simulink model "dynamicCalibrationDataGenerator"  (R2022b)
settings: Solver=VariableStepAuto  StartTime=0.0  StopTime=20  RelTol=1e-3
values from neighbouring files (symbols this model uses):
  acc_bias = [2*(rand-0.5)*acc_xy_bias_tolerance 2*(rand-0.5)*acc_xy_bias_tolerance 2*(rand-0.5)*acc_z_bias_tolerance]    [sim_cfg.m]
  acc_bias_over_temp = 2*(rand([1 3])-0.5)*acc_bias_over_temp_tolerance    [sim_cfg.m]
  acc_dynamic = 2*9.81    (= 19.62)    [sim_cfg.m]
  acc_freq = 100    [sim_cfg.m]
  acc_gain_over_temp = diag(2*(rand([1 3])-0.5)*acc_bias_over_temp_tolerance)    [sim_cfg.m]
  acc_noise = 0.008*9.81    (= 0.07848)    [sim_cfg.m]
  acc_non_orthogonality = acc_axis_alignement*acc_non_orthogonality    [sim_cfg.m]
  f_sim = 100    [sim_cfg.m]
  gps_freq = 20    [sim_cfg.m]
  gps_xy_noise = 0.1    [sim_cfg.m]
  gps_z_noise = 0.1    [sim_cfg.m]
  gravity = 9.81+rand()*0.005    [sim_cfg.m]
  gyr_bias = 2*(rand([1 3])-0.5)*gyr_bias_tolerance    [sim_cfg.m]
  gyr_bias_over_temp = 2*(rand([1 3])-0.5)*gyr_bias_over_temp_tolerance    [sim_cfg.m]
  gyr_dynamic = 250*pi/180    (= 4.36332312999)    [sim_cfg.m]
  gyr_freq = 100    [sim_cfg.m]
  gyr_gain_over_temp = diag(2*(rand([1 3])-0.5)*gyr_bias_over_temp_tolerance)    [sim_cfg.m]
  gyr_noise = 0.1*pi/180    (= 0.00174532925199)    [sim_cfg.m]
  gyr_non_orthogonality = gyr_axis_alignement*gyr_non_orthogonality    [sim_cfg.m]
  random_move_power = 3    [sim_cfg.m]
  temp_dynamic = 1    [sim_cfg.m]
libraries: simulink x10
settings Model: Creator=student  LastModifiedBy=robin

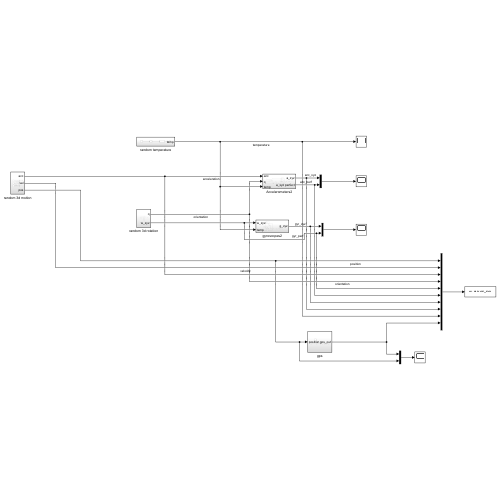
[thumbnail: Simulink's stored preview of the top-level diagram]
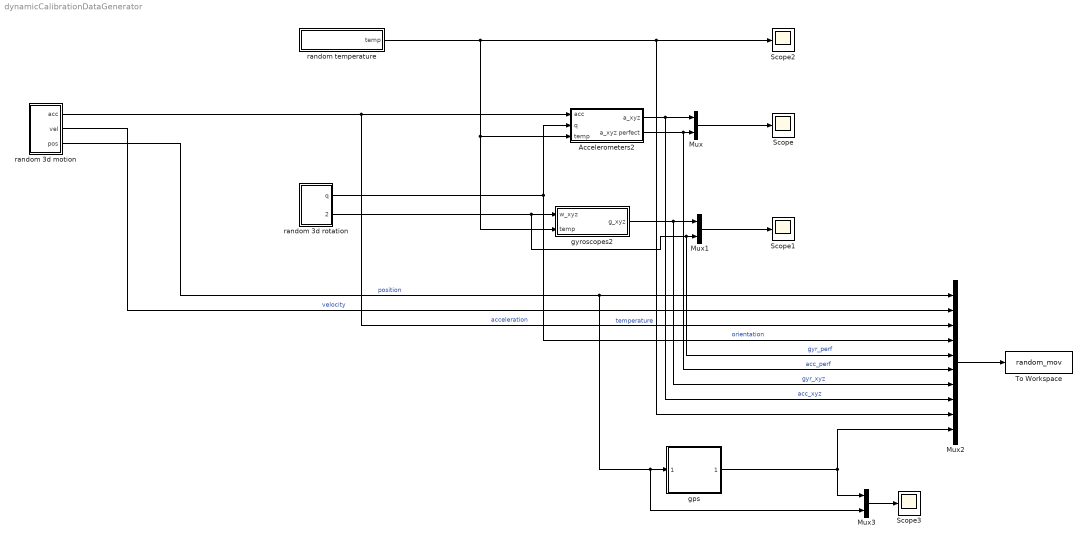
== system dynamicCalibrationDataGenerator ==
  Accelerometers2 : Subsystem
  Mux : Mux  Inputs=2
  Mux1 : Mux  Inputs=2
  Mux2 : Mux  Inputs=10
  Mux3 : Mux  Inputs=2
  Scope{,1..3} (4 alike) : Scope
  To Workspace : ToWorkspace  VariableName=random_mov  SaveFormat=Structure With Time  SampleTime=1/f_sim
  gps : Subsystem
  gyroscopes2 : Subsystem
  random 3d motion : Subsystem
  random 3d rotation : Subsystem
  random temperature : Subsystem
  wires:
  random 3d motion/1(acc) -> Accelerometers2/1(acc), Mux2/3  "acceleration"
  random 3d rotation/1(q) -> Accelerometers2/2(q), Mux2/4  "orientation"
  random 3d rotation/2(w_xyz) -> gyroscopes2/1(w_xyz), Mux2/5, Mux1/2  "gyr_perf"
  gyroscopes2/1(g_xyz) -> Mux2/7, Mux1/1  "gyr_xyz"
  random temperature/1(temp) -> gyroscopes2/2(temp), Accelerometers2/3(temp), Scope2/1, Mux2/9  "temperature"
  Accelerometers2/1(a_xyz) -> Mux2/8, Mux/1  "acc_xyz"
  Accelerometers2/2(a_xyz perfect) -> Mux2/6, Mux/2  "acc_perf"
  Mux/1 -> Scope/1
  Mux1/1 -> Scope1/1
  random 3d motion/3(pos) -> Mux3/2, gps/1(position), Mux2/1  "position"
  random 3d motion/2(vel) -> Mux2/2  "velocity"
  Mux2/1 -> To Workspace/1
  gps/1(gps_out) -> Mux3/1, Mux2/10
  Mux3/1 -> Scope3/1

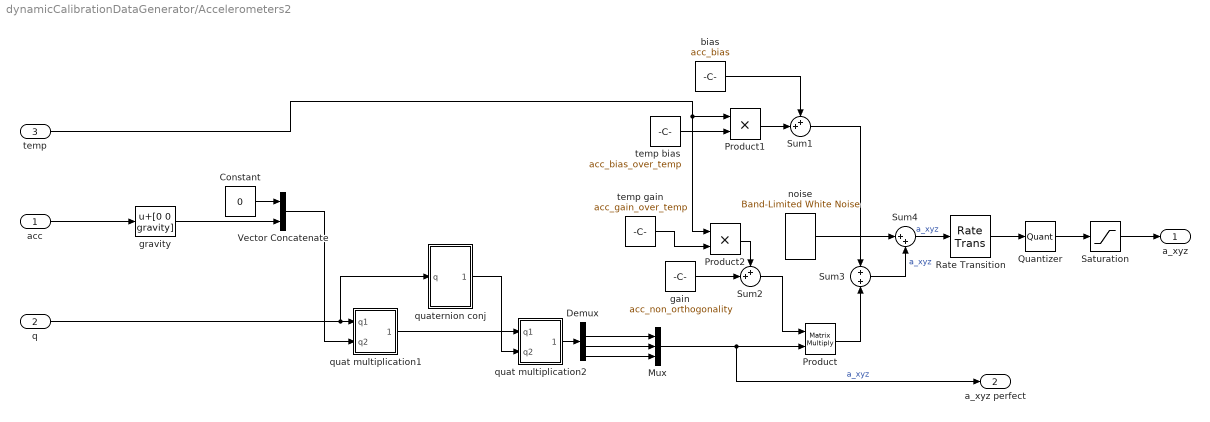
== system dynamicCalibrationDataGenerator/Accelerometers2 ==
  acc : Inport
  q : Inport  Port=2
  temp : Inport  Port=3
  Constant : Constant  Value=0
  Demux : Demux
  Mux : Mux  Inputs=3
  Product : Product  Multiplication=Matrix(*)
  Product1 : Product
  Product2 : Product
  Quantizer : Quantizer  QuantizationInterval=acc_res
  Rate Transition : RateTransition  OutPortSampleTime=1/acc_freq
  Saturation : Saturate  UpperLimit=acc_dynamic  LowerLimit=-acc_dynamic
  Sum1 : Sum  Inputs=++|
  Sum2 : Sum  Inputs=++|
  Sum3 : Sum
  Sum4 : Sum  Inputs=|++
  Vector Concatenate : Concatenate
  bias : Constant  Value=acc_bias
  gain : Constant  Value=acc_non_orthogonality
  gravity : Bias  Bias=[0 0 gravity]  SaturateOnIntegerOverflow=off
  noise : simulink/Sources/Band-Limited White Noise  Cov=[2*(2*pi*acc_noise/acc_freq)^2 2*(2*pi*acc_noise/acc_freq)^2 2*(2*pi*acc_noise/acc_freq)^2]  Ts=1/acc_freq  seed=[randi(10000) randi(10000) randi(10000)]  VectorParams1D=off
  quat multiplication1 : Subsystem
  quat multiplication2 : Subsystem
  quaternion conj : Subsystem
  temp bias : Constant  Value=acc_bias_over_temp
  temp gain : Constant  Value=acc_gain_over_temp
  a_xyz : Outport
  a_xyz perfect : Outport  Port=2
  wires:
  q/1 -> quat multiplication1/1(q1), quaternion conj/1(q)
  Sum4/1 -> Rate Transition/1  "a_xyz"
  Constant/1 -> Vector Concatenate/1
  Vector Concatenate/1 -> quat multiplication1/2(q2)
  gravity/1 -> Vector Concatenate/2
  quaternion conj/1(q conj) -> quat multiplication2/2(q2)
  quat multiplication1/1(q1*q2) -> quat multiplication2/1(q1)
  acc/1 -> gravity/1
  quat multiplication2/1(q1*q2) -> Demux/1
  Demux/2 -> Mux/1
  Demux/3 -> Mux/2
  Demux/4 -> Mux/3
  bias/1 -> Sum1/1
  Product1/1 -> Sum1/2
  temp bias/1 -> Product1/2
  temp/1 -> Product2/1, Product1/1
  temp gain/1 -> Product2/2
  gain/1 -> Sum2/2
  Sum2/1 -> Product/1
  Product2/1 -> Sum2/1
  Product/1 -> Sum3/2
  Sum1/1 -> Sum3/1
  Sum3/1 -> Sum4/2  "a_xyz"
  noise/1 -> Sum4/1
  Mux/1 -> a_xyz perfect/1, Product/2  "a_xyz"
  Saturation/1 -> a_xyz/1
  Rate Transition/1 -> Quantizer/1
  Quantizer/1 -> Saturation/1

== system dynamicCalibrationDataGenerator/gps ==
  position : Inport
  Band-Limited White Noise1 : simulink/Sources/Band-Limited White Noise  Cov=[2*(2*pi*gps_xy_noise/gps_freq)^2 2*(2*pi*gps_xy_noise/gps_freq)^2 2*(2*pi*gps_z_noise/gps_freq)^2]  Ts=1/gps_freq  seed=[randi(10000) randi(10000) randi(10000)]  VectorParams1D=off
  Quantizer : Quantizer  QuantizationInterval=gps_res
  Rate Transition : RateTransition  OutPortSampleTime=1/gps_freq
  Sum3 : Sum  Inputs=++|
  gps_out : Outport
  wires:
  Rate Transition/1 -> Quantizer/1
  Quantizer/1 -> gps_out/1
  Band-Limited White Noise1/1 -> Sum3/1
  Sum3/1 -> Rate Transition/1
  position/1 -> Sum3/2

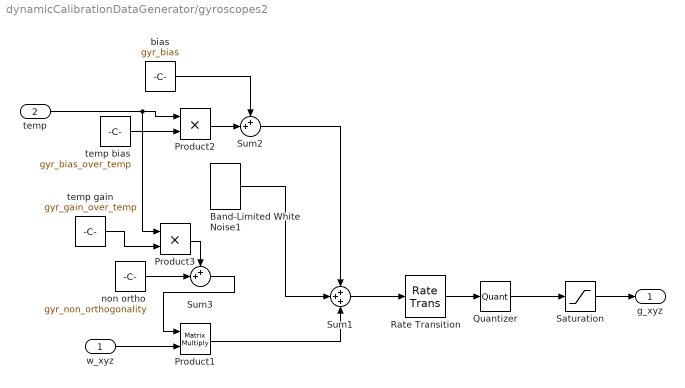
== system dynamicCalibrationDataGenerator/gyroscopes2 ==
  w_xyz : Inport
  temp : Inport  Port=2
  Band-Limited White Noise1 : simulink/Sources/Band-Limited White Noise  Cov=[2*(2*pi*gyr_noise/gyr_freq)^2 2*(2*pi*gyr_noise/gyr_freq)^2 2*(2*pi*gyr_noise/gyr_freq)^2]  Ts=1/gyr_freq  seed=[randi(10000) randi(10000) randi(10000)]  VectorParams1D=off
  Product1 : Product  Multiplication=Matrix(*)
  Product2 : Product
  Product3 : Product
  Quantizer : Quantizer  QuantizationInterval=gyr_res
  Rate Transition : RateTransition  OutPortSampleTime=1/gyr_freq
  Saturation : Saturate  UpperLimit=gyr_dynamic  LowerLimit=-gyr_dynamic
  Sum1 : Sum  Inputs=+++
  Sum2 : Sum  Inputs=++|
  Sum3 : Sum  Inputs=++|
  bias : Constant  Value=gyr_bias
  non ortho : Constant  Value=gyr_non_orthogonality
  temp bias : Constant  Value=gyr_bias_over_temp
  temp gain : Constant  Value=gyr_gain_over_temp
  g_xyz : Outport
  wires:
  non ortho/1 -> Sum3/2
  Product3/1 -> Sum3/1
  temp/1 -> Product3/1, Product2/1
  Product2/1 -> Sum2/2
  temp gain/1 -> Product3/2
  temp bias/1 -> Product2/2
  Sum3/1 -> Product1/1
  bias/1 -> Sum2/1
  Band-Limited White Noise1/1 -> Sum1/2
  Sum2/1 -> Sum1/1
  w_xyz/1 -> Product1/2
  Product1/1 -> Sum1/3
  Saturation/1 -> g_xyz/1
  Rate Transition/1 -> Quantizer/1
  Sum1/1 -> Rate Transition/1
  Quantizer/1 -> Saturation/1

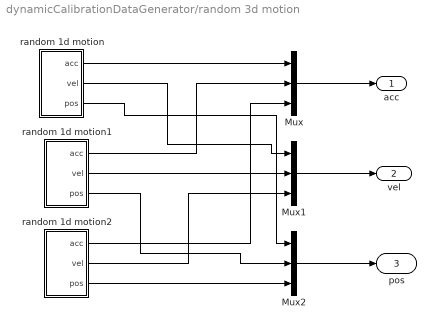
== system dynamicCalibrationDataGenerator/random 3d motion ==
  Mux : Mux  Inputs=3
  Mux1 : Mux  Inputs=3
  Mux2 : Mux  Inputs=3
  random 1d motion : Subsystem
  random 1d motion1 : Subsystem
  random 1d motion2 : Subsystem
  acc : Outport
  vel : Outport  Port=2
  pos : Outport  Port=3
  wires:
  random 1d motion/2(vel) -> Mux1/1
  random 1d motion1/3(pos) -> Mux2/2
  random 1d motion1/2(vel) -> Mux1/2
  Mux/1 -> acc/1
  random 1d motion/3(pos) -> Mux2/1
  random 1d motion2/3(pos) -> Mux2/3
  random 1d motion2/2(vel) -> Mux1/3
  random 1d motion2/1(acc) -> Mux/3
  random 1d motion/1(acc) -> Mux/1
  random 1d motion1/1(acc) -> Mux/2
  Mux1/1 -> vel/1
  Mux2/1 -> pos/1

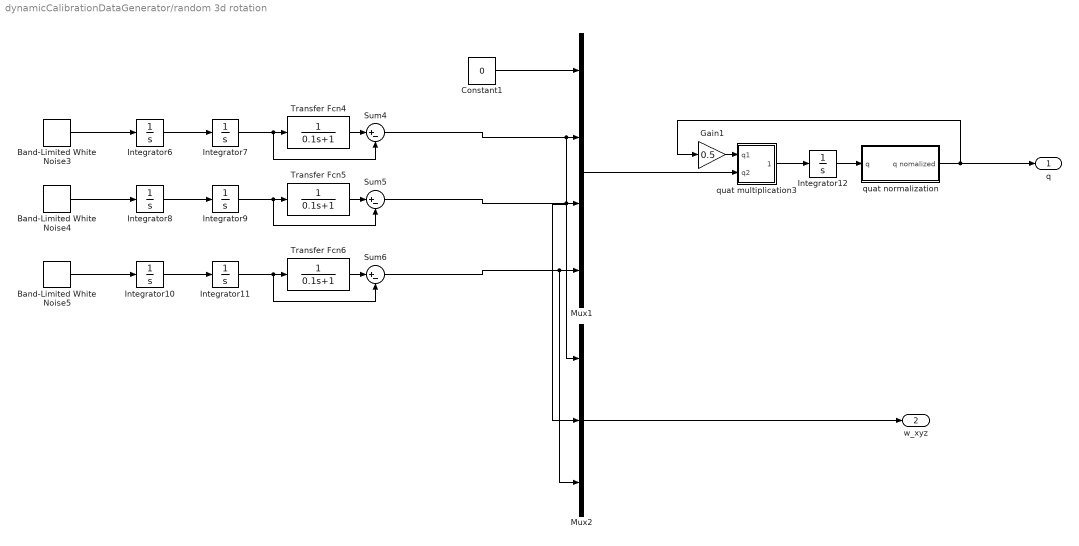
== system dynamicCalibrationDataGenerator/random 3d rotation ==
  Band-Limited White Noise3 : simulink/Sources/Band-Limited White Noise  Cov=[1]  Ts=0.1  seed=[randi(10000)]
  Band-Limited White Noise4 : simulink/Sources/Band-Limited White Noise  Cov=[1]  Ts=0.1  seed=[randi(10000)]
  Band-Limited White Noise5 : simulink/Sources/Band-Limited White Noise  Cov=[1]  Ts=0.1  seed=[randi(10000)]
  Constant1 : Constant  Value=0
  Gain1 : Gain  Gain=0.5
  Integrator{6..11} (6 alike) : Integrator
  Integrator12 : Integrator  InitialCondition=[1 0 0 0]
  Mux1 : Mux
  Mux2 : Mux  Inputs=3
  Sum4 : Sum  Inputs=|+-
  Sum5 : Sum  Inputs=|+-
  Sum6 : Sum  Inputs=|+-
  Transfer Fcn4 : TransferFcn  Denominator=[0.1 1]
  Transfer Fcn5 : TransferFcn  Denominator=[0.1 1]
  Transfer Fcn6 : TransferFcn  Denominator=[0.1 1]
  quat multiplication3 : Subsystem
  quat normalization : Subsystem
  q : Outport
  w_xyz : Outport  Port=2
  wires:
  Sum6/1 -> Mux1/4, Mux2/3
  Gain1/1 -> quat multiplication3/1(q1)
  Constant1/1 -> Mux1/1
  Mux2/1 -> w_xyz/1
  Sum4/1 -> Mux2/1, Mux1/2
  Integrator12/1 -> quat normalization/1(q)
  Sum5/1 -> Mux2/2, Mux1/3
  Integrator6/1 -> Integrator7/1
  Transfer Fcn6/1 -> Sum6/1
  Band-Limited White Noise4/1 -> Integrator8/1
  Integrator10/1 -> Integrator11/1
  Integrator7/1 -> Sum4/2, Transfer Fcn4/1
  Band-Limited White Noise5/1 -> Integrator10/1
  Integrator11/1 -> Sum6/2, Transfer Fcn6/1
  Mux1/1 -> quat multiplication3/2(q2)
  Integrator8/1 -> Integrator9/1
  Band-Limited White Noise3/1 -> Integrator6/1
  Integrator9/1 -> Sum5/2, Transfer Fcn5/1
  Transfer Fcn4/1 -> Sum4/1
  Transfer Fcn5/1 -> Sum5/1
  quat multiplication3/1(q1*q2) -> Integrator12/1
  quat normalization/1(q nomalized) -> Gain1/1, q/1

== system dynamicCalibrationDataGenerator/random temperature ==
  Band-Limited White Noise : simulink/Sources/Band-Limited White Noise  Cov=[1]  Ts=0.1  seed=[randi(10000)]
  Integrator Limited : Integrator  LimitOutput=on  UpperSaturationLimit=temp_dynamic/2  LowerSaturationLimit=-temp_dynamic/2
  Transfer Fcn1 : TransferFcn  Denominator=[0.1 1]
  temp : Outport
  wires:
  Band-Limited White Noise/1 -> Integrator Limited/1
  Transfer Fcn1/1 -> temp/1
  Integrator Limited/1 -> Transfer Fcn1/1

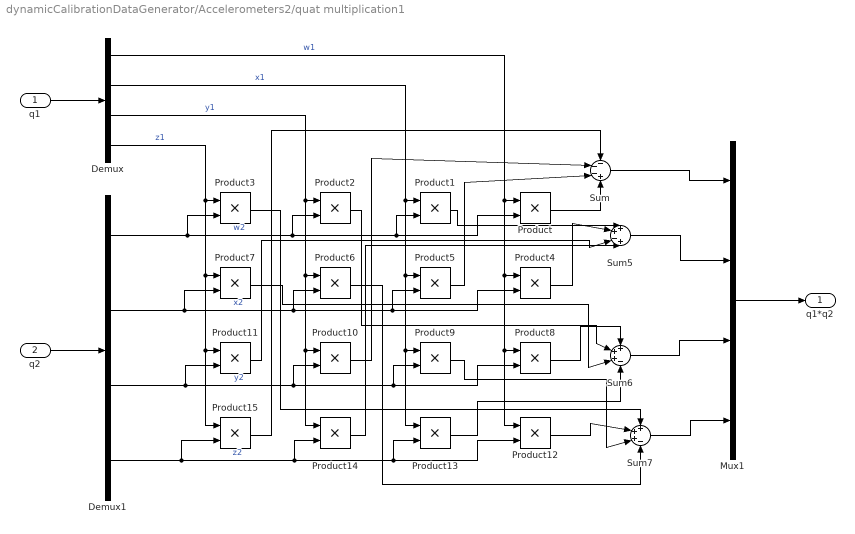
== system dynamicCalibrationDataGenerator/Accelerometers2/quat multiplication1 ==
  q1 : Inport
  q2 : Inport  Port=2
  Demux : Demux
  Demux1 : Demux
  Mux1 : Mux
  Product{,1..15} (16 alike) : Product
  Sum : Sum  Inputs=---+
  Sum5 : Sum  Inputs=++-+
  Sum6 : Sum  Inputs=+++-
  Sum7 : Sum  Inputs=+++-
  q1*q2 : Outport
  wires:
  Sum5/1 -> Mux1/2
  Product/1 -> Sum/4
  Product9/1 -> Sum7/3
  Demux/1 -> Product12/1, Product8/1, Product4/1, Product/1  "w1"
  Demux1/3 -> Product8/2, Product9/2, Product10/2, Product11/2  "y2"
  Demux/2 -> Product13/1, Product9/1, Product5/1, Product1/1  "x1"
  Product6/1 -> Sum7/4
  Product4/1 -> Sum5/2
  Demux1/1 -> Product/2, Product1/2, Product2/2, Product3/2  "w2"
  Sum/1 -> Mux1/1
  Product3/1 -> Sum7/1
  Product15/1 -> Sum/1
  Product1/1 -> Sum5/1
  Product2/1 -> Sum6/2
  Demux/4 -> Product15/1, Product11/1, Product7/1, Product3/1  "z1"
  Sum6/1 -> Mux1/3
  Demux1/2 -> Product4/2, Product5/2, Product6/2, Product7/2  "x2"
  Demux1/4 -> Product12/2, Product13/2, Product14/2, Product15/2  "z2"
  Product14/1 -> Sum5/4
  Mux1/1 -> q1*q2/1
  Sum7/1 -> Mux1/4
  Demux/3 -> Product14/1, Product10/1, Product6/1, Product2/1  "y1"
  Product13/1 -> Sum6/4
  Product8/1 -> Sum6/1
  q2/1 -> Demux1/1
  q1/1 -> Demux/1
  Product11/1 -> Sum5/3
  Product7/1 -> Sum6/3
  Product10/1 -> Sum/2
  Product5/1 -> Sum/3
  Product12/1 -> Sum7/2

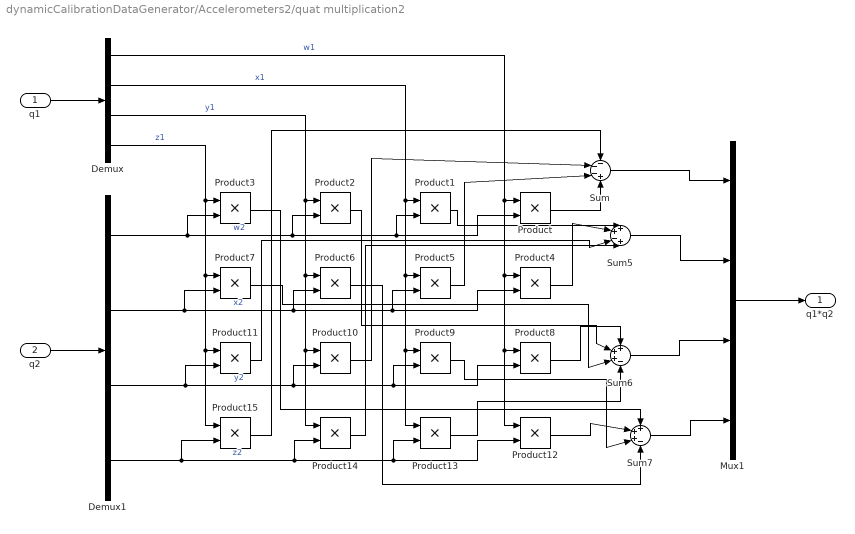
== system dynamicCalibrationDataGenerator/Accelerometers2/quat multiplication2 ==
  q1 : Inport
  q2 : Inport  Port=2
  Demux : Demux
  Demux1 : Demux
  Mux1 : Mux
  Product{,1..15} (16 alike) : Product
  Sum : Sum  Inputs=---+
  Sum5 : Sum  Inputs=++-+
  Sum6 : Sum  Inputs=+++-
  Sum7 : Sum  Inputs=+++-
  q1*q2 : Outport
  wires:
  Sum5/1 -> Mux1/2
  Product/1 -> Sum/4
  Product9/1 -> Sum7/3
  Demux/1 -> Product12/1, Product8/1, Product4/1, Product/1  "w1"
  Demux1/3 -> Product8/2, Product9/2, Product10/2, Product11/2  "y2"
  Demux/2 -> Product13/1, Product9/1, Product5/1, Product1/1  "x1"
  Product6/1 -> Sum7/4
  Product4/1 -> Sum5/2
  Demux1/1 -> Product/2, Product1/2, Product2/2, Product3/2  "w2"
  Sum/1 -> Mux1/1
  Product3/1 -> Sum7/1
  Product15/1 -> Sum/1
  Product1/1 -> Sum5/1
  Product2/1 -> Sum6/2
  Demux/4 -> Product15/1, Product11/1, Product7/1, Product3/1  "z1"
  Sum6/1 -> Mux1/3
  Demux1/2 -> Product4/2, Product5/2, Product6/2, Product7/2  "x2"
  Demux1/4 -> Product12/2, Product13/2, Product14/2, Product15/2  "z2"
  Product14/1 -> Sum5/4
  Mux1/1 -> q1*q2/1
  Sum7/1 -> Mux1/4
  Demux/3 -> Product14/1, Product10/1, Product6/1, Product2/1  "y1"
  Product13/1 -> Sum6/4
  Product8/1 -> Sum6/1
  q2/1 -> Demux1/1
  q1/1 -> Demux/1
  Product11/1 -> Sum5/3
  Product7/1 -> Sum6/3
  Product10/1 -> Sum/2
  Product5/1 -> Sum/3
  Product12/1 -> Sum7/2

== system dynamicCalibrationDataGenerator/Accelerometers2/quaternion conj ==
  q : Inport
  Demux : Demux
  Gain : Gain  Gain=-1
  Gain2 : Gain  Gain=-1
  Gain3 : Gain  Gain=-1
  Mux : Mux
  q conj : Outport
  wires:
  Gain2/1 -> Mux/3
  Demux/3 -> Gain2/1  "y1"
  Demux/1 -> Mux/1  "w1"
  Gain3/1 -> Mux/4
  Demux/4 -> Gain3/1  "z1"
  q/1 -> Demux/1
  Mux/1 -> q conj/1
  Demux/2 -> Gain/1  "x1"
  Gain/1 -> Mux/2

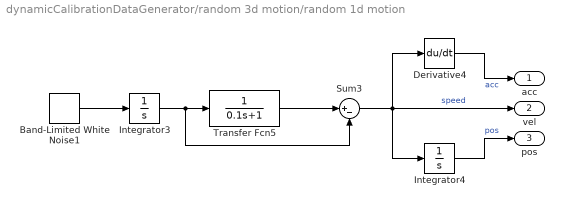
== system dynamicCalibrationDataGenerator/random 3d motion/random 1d motion ==
  Band-Limited White Noise1 : simulink/Sources/Band-Limited White Noise  Cov=[random_move_power]  Ts=0.1  seed=[randi(10000)]
  Derivative4 : Derivative
  Integrator3 : Integrator
  Integrator4 : Integrator
  Sum3 : Sum  Inputs=|+-
  Transfer Fcn5 : TransferFcn  Denominator=[0.1 1]
  acc : Outport
  vel : Outport  Port=2
  pos : Outport  Port=3
  wires:
  Band-Limited White Noise1/1 -> Integrator3/1
  Integrator3/1 -> Transfer Fcn5/1, Sum3/2
  Transfer Fcn5/1 -> Sum3/1
  Sum3/1 -> vel/1, Integrator4/1, Derivative4/1  "speed"
  Derivative4/1 -> acc/1  "acc"
  Integrator4/1 -> pos/1  "pos"

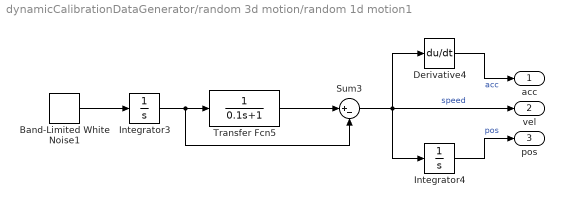
== system dynamicCalibrationDataGenerator/random 3d motion/random 1d motion1 ==
  Band-Limited White Noise1 : simulink/Sources/Band-Limited White Noise  Cov=[random_move_power]  Ts=0.1  seed=[randi(10000)]
  Derivative4 : Derivative
  Integrator3 : Integrator
  Integrator4 : Integrator
  Sum3 : Sum  Inputs=|+-
  Transfer Fcn5 : TransferFcn  Denominator=[0.1 1]
  acc : Outport
  vel : Outport  Port=2
  pos : Outport  Port=3
  wires:
  Band-Limited White Noise1/1 -> Integrator3/1
  Integrator3/1 -> Transfer Fcn5/1, Sum3/2
  Transfer Fcn5/1 -> Sum3/1
  Sum3/1 -> vel/1, Integrator4/1, Derivative4/1  "speed"
  Derivative4/1 -> acc/1  "acc"
  Integrator4/1 -> pos/1  "pos"

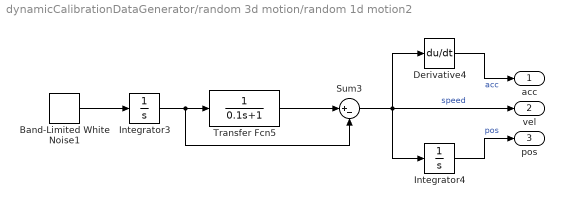
== system dynamicCalibrationDataGenerator/random 3d motion/random 1d motion2 ==
  Band-Limited White Noise1 : simulink/Sources/Band-Limited White Noise  Cov=[random_move_power]  Ts=0.1  seed=[randi(10000)]
  Derivative4 : Derivative
  Integrator3 : Integrator
  Integrator4 : Integrator
  Sum3 : Sum  Inputs=|+-
  Transfer Fcn5 : TransferFcn  Denominator=[0.1 1]
  acc : Outport
  vel : Outport  Port=2
  pos : Outport  Port=3
  wires:
  Band-Limited White Noise1/1 -> Integrator3/1
  Integrator3/1 -> Transfer Fcn5/1, Sum3/2
  Transfer Fcn5/1 -> Sum3/1
  Sum3/1 -> vel/1, Integrator4/1, Derivative4/1  "speed"
  Derivative4/1 -> acc/1  "acc"
  Integrator4/1 -> pos/1  "pos"

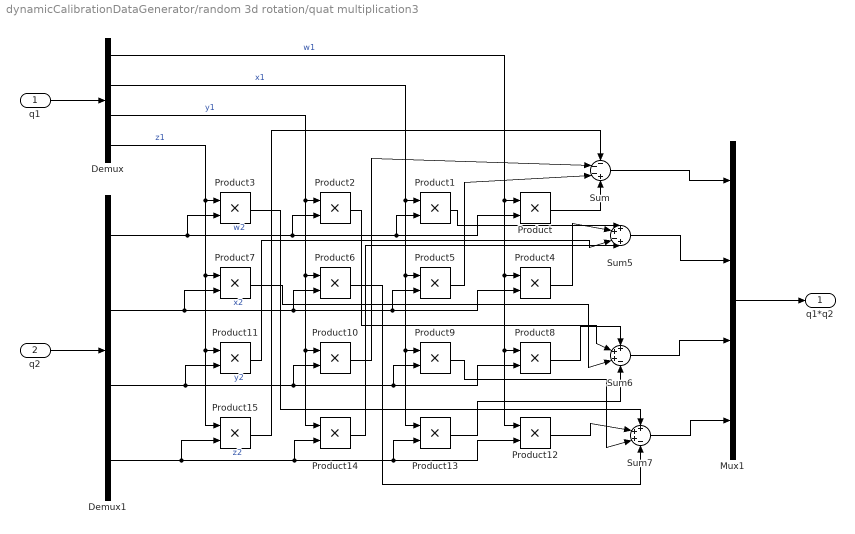
== system dynamicCalibrationDataGenerator/random 3d rotation/quat multiplication3 ==
  q1 : Inport
  q2 : Inport  Port=2
  Demux : Demux
  Demux1 : Demux
  Mux1 : Mux
  Product{,1..15} (16 alike) : Product
  Sum : Sum  Inputs=---+
  Sum5 : Sum  Inputs=++-+
  Sum6 : Sum  Inputs=+++-
  Sum7 : Sum  Inputs=+++-
  q1*q2 : Outport
  wires:
  Sum5/1 -> Mux1/2
  Product/1 -> Sum/4
  Product9/1 -> Sum7/3
  Demux/1 -> Product12/1, Product8/1, Product4/1, Product/1  "w1"
  Demux1/3 -> Product8/2, Product9/2, Product10/2, Product11/2  "y2"
  Demux/2 -> Product13/1, Product9/1, Product5/1, Product1/1  "x1"
  Product6/1 -> Sum7/4
  Product4/1 -> Sum5/2
  Demux1/1 -> Product/2, Product1/2, Product2/2, Product3/2  "w2"
  Sum/1 -> Mux1/1
  Product3/1 -> Sum7/1
  Product15/1 -> Sum/1
  Product1/1 -> Sum5/1
  Product2/1 -> Sum6/2
  Demux/4 -> Product15/1, Product11/1, Product7/1, Product3/1  "z1"
  Sum6/1 -> Mux1/3
  Demux1/2 -> Product4/2, Product5/2, Product6/2, Product7/2  "x2"
  Demux1/4 -> Product12/2, Product13/2, Product14/2, Product15/2  "z2"
  Product14/1 -> Sum5/4
  Mux1/1 -> q1*q2/1
  Sum7/1 -> Mux1/4
  Demux/3 -> Product14/1, Product10/1, Product6/1, Product2/1  "y1"
  Product13/1 -> Sum6/4
  Product8/1 -> Sum6/1
  q2/1 -> Demux1/1
  q1/1 -> Demux/1
  Product11/1 -> Sum5/3
  Product7/1 -> Sum6/3
  Product10/1 -> Sum/2
  Product5/1 -> Sum/3
  Product12/1 -> Sum7/2

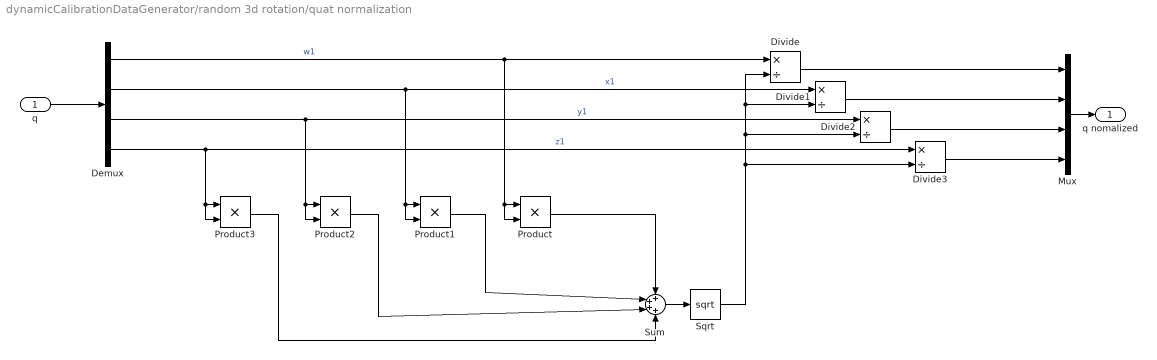
== system dynamicCalibrationDataGenerator/random 3d rotation/quat normalization ==
  q : Inport
  Demux : Demux
  Divide{,1..3} (4 alike) : Product  Inputs=*/
  Mux : Mux
  Product{,1..3} (4 alike) : Product
  Sqrt : Sqrt
  Sum : Sum  Inputs=++++
  q nomalized : Outport
  wires:
  Demux/1 -> Product/2, Product/1, Divide/1  "w1"
  Demux/2 -> Product1/2, Product1/1, Divide1/1  "x1"
  Demux/4 -> Product3/2, Product3/1, Divide3/1  "z1"
  Demux/3 -> Product2/2, Product2/1, Divide2/1  "y1"
  q/1 -> Demux/1
  Product/1 -> Sum/1
  Product1/1 -> Sum/2
  Product2/1 -> Sum/3
  Product3/1 -> Sum/4
  Sum/1 -> Sqrt/1
  Sqrt/1 -> Divide3/2, Divide2/2, Divide1/2, Divide/2
  Divide3/1 -> Mux/4
  Divide2/1 -> Mux/3
  Divide1/1 -> Mux/2
  Divide/1 -> Mux/1
  Mux/1 -> q nomalized/1
